simulink model "yarpReadDoubles"  (Simulink 7.3)
settings: Solver=ode45  SolverMode=SingleTasking  StartTime=0.0  StopTime=inf  RelTol=1e-3  AbsTol=1e-6
libraries: utility x1
settings Model: Creator=dmedonza  LastModifiedBy=yo
settings DataIOCC: SaveOutput=off  SignalLogging=off  SaveTime=off
settings OptimizationCC: BooleanDataType=off
settings DebuggingCC: SaveWithParameterizedLinksMsg=none  SignalResolutionControl=TryResolveAllWithWarning  SolverPrmCheckMsg=none  MultiTaskDSMMsg=warning  MultiTaskCondExecSysMsg=none  StrictBusMsg=None
settings HardwareCC: TargetUnknown=on
settings RTWCC: TemplateMakefile=grt_vc.tmf  IncludeERTFirstTime=on

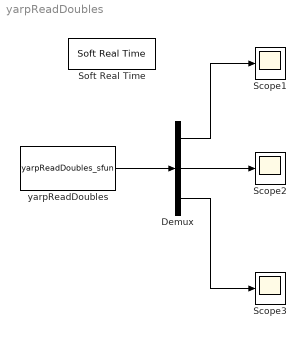
== system yarpReadDoubles ==
  Demux : Demux  Outputs=3
  Scope1 : Scope
      settings: TimeRange=10  YMin=0  YMax=25
  Scope2 : Scope
      settings: YMin=0  YMax=20
  Scope3 : Scope
      settings: YMin=0  YMax=3  SaveName=ScopeData2
  Soft Real Time : utility/Soft Real Time  x=1
  yarpReadDoubles : S-Function  FunctionName=yarpReadDoubles_sfun  Parameters=setNumDoubles  EnableBusSupport=off  mask{setNumDoubles=3}
      mask prompts: setNumDoubles "Number of Doubles"
      mask help: The yarpWriteDoubles block tries to open a YARP port called /yarpReadDoubles, connect from a port called /write, and then read some streaming doubles!!!
      mask Display: image(imread('yarpPipes.png'))
  wires:
  Demux/1 -> Scope1/1
  Demux/2 -> Scope2/1
  Demux/3 -> Scope3/1
  yarpReadDoubles/1 -> Demux/1
